simulink model "alt_dspbuilder_internal_InitializedRegister"  (Simulink 6.6)
settings: Solver=ode45  StartTime=0.0  StopTime=10.0  RelTol=1e-3
InitFcn:
  | %% DSPBuilder Start
  | alt_dspbuilder_update_model(bdroot)
  | %% DSPBuilder End
libraries: allblocks_alteradspbuilder2 x8
settings Model: Creator=cpurcell  LastModifiedBy=mjervis
settings DebuggingCC: AlgebraicLoopMsg=none  SignalResolutionControl=TryResolveAllWithWarning  MultiTaskDSMMsg=warning  MultiTaskCondExecSysMsg=none
settings RTWCC: IncludeERTFirstTime=on

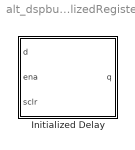
== system alt_dspbuilder_internal_InitializedRegister ==
  Initialized Delay : Subsystem  mask(Initialized Register AlteraBlockSet){sgn=Signed Integer, bwl=8, bwr=0, reset_value=1}
      mask prompts: sgn "Data Type"; bwl "[Number Of Bits].[]"; bwr "[].[Number Of Bits]"; reset_value "Reset Value"
      mask help:
      | Implements a register with an initialization value.
      |
      | Inputs:
      | d - data input
      | ena - Enable
      | aclr - Asynchronous clear
      |
      | Outputs:
      | q - Data out
      mask init:
      | alt_dspbuilder_internal_InitializedRegister_Init(gcb,1,1,bwl,bwr,reset_value);
      mask Help: helpview(fullfile(alt_dspbuilder_get_quartus_rootdir, 'dsp_builder', 'docs', 'InitializedRegister.html'))
      mask StyleString: popup(Signed Integer|Signed Fractional|Unsigned Integer),edit,edit,edit
      mask CallbackString: alt_dspbuilder_internal_InitializedRegister_Init(gcb,1,0);|alt_dspbuilder_internal_InitializedRegister_Init(gcb,1,0);|alt_dspbuilder_internal_InitializedRegister_Init(gcb,1,0);|alt_dspbuilder_internal_InitializedRegister_Init(gcb,1,0);

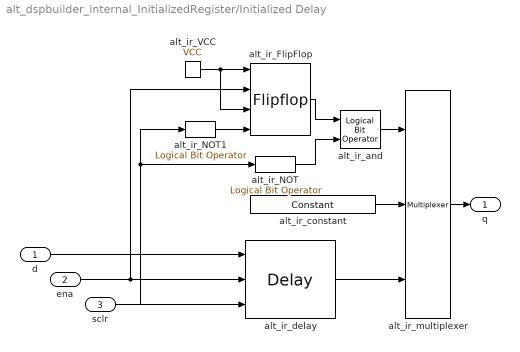
== system alt_dspbuilder_internal_InitializedRegister/Initialized Delay ==
  d : Inport
  ena : Inport  Port=2
  sclr : Inport  Port=3
  alt_ir_FlipFlop : allblocks_alteradspbuilder2/Flipflop  mode=DFFE  BusType=Signed Fractional  bwl=1  bwr=1
  alt_ir_NOT : allblocks_alteradspbuilder2/Logical Bit Operator  LogicalOperator=NOT  user_inputs=2
  alt_ir_NOT1 : allblocks_alteradspbuilder2/Logical Bit Operator  LogicalOperator=NOT  user_inputs=2
  alt_ir_VCC : allblocks_alteradspbuilder2/VCC  SpecifyClock=off
  alt_ir_and : allblocks_alteradspbuilder2/Logical Bit Operator  LogicalOperator=AND  user_inputs=2
  alt_ir_constant : allblocks_alteradspbuilder2/Constant  mask_cst=reset_value  BusType=Signed Integer  bwl=bwl  bwr=bwr  SpecifyClock=off
  alt_ir_delay : allblocks_alteradspbuilder2/Delay  pipeline=1  ClockPhase=1  use_ena=on  use_sclr=on
  alt_ir_multiplexer : allblocks_alteradspbuilder2/Multiplexer  numInputs=2  pipeline=1  oneHot=off  use_ena=off  use_aclr=off
  q : Outport
  wires:
  alt_ir_multiplexer/1 -> q/1
  alt_ir_VCC/1 -> alt_ir_FlipFlop/3, alt_ir_FlipFlop/1
  alt_ir_constant/1 -> alt_ir_multiplexer/2
  alt_ir_FlipFlop/1 -> alt_ir_and/1
  alt_ir_and/1 -> alt_ir_multiplexer/1
  alt_ir_NOT/1 -> alt_ir_and/2
  alt_ir_NOT1/1 -> alt_ir_FlipFlop/4
  alt_ir_delay/1 -> alt_ir_multiplexer/3
  ena/1 -> alt_ir_FlipFlop/2, alt_ir_delay/2
  sclr/1 -> alt_ir_NOT/1, alt_ir_delay/3, alt_ir_NOT1/1
  d/1 -> alt_ir_delay/1
